simulink model "RCAM_OP_LONG_AP_SM_CL_FULL"  (R2022b)
settings: Solver=VariableStepAuto  StartTime=0.0  StopTime=100.0  RelTol=1e-3
undefined symbols (not defined in the file): H_nz, K_nzq
libraries: cstblocks x1
settings Model: Creator=bendr  LastModifiedBy=bendr

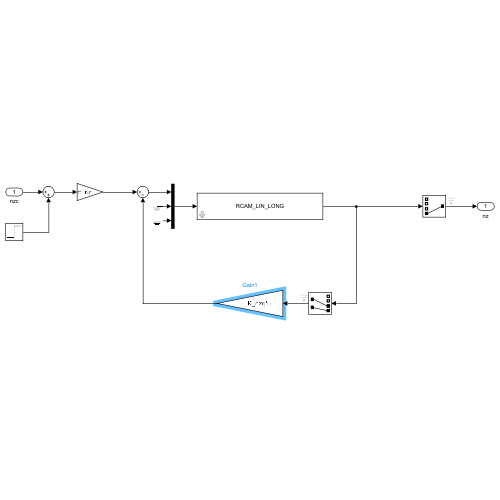
[thumbnail: Simulink's stored preview of the top-level diagram]
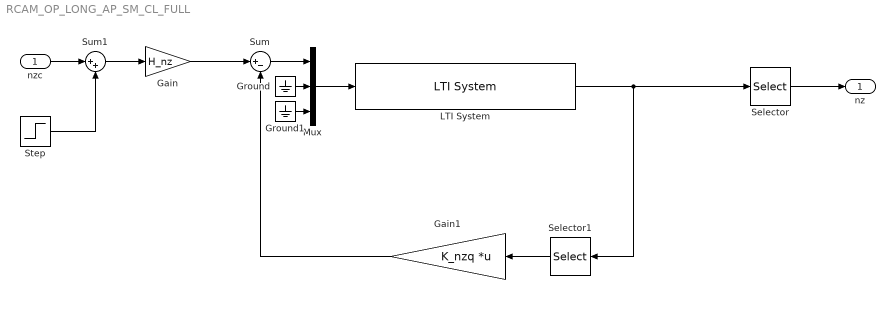
== system RCAM_OP_LONG_AP_SM_CL_FULL ==
  nzc : Inport
  Gain : Gain  Gain=H_nz
  Gain1 : Gain  Gain=K_nzq  Multiplication=Matrix(K*u)
  Ground : Ground
  Ground1 : Ground
  LTI System : cstblocks/LTI System  sys=RCAM_LIN_LONG  IC=[]
  Mux : Mux  Inputs=3
  Selector : Selector  InputPortWidth=4  IndexOptions=Index vector (dialog)  Indices=4  OutputSizes=1
  Selector1 : Selector  InputPortWidth=4  IndexOptions=Index vector (dialog)  Indices=[3 4]  OutputSizes=1
  Step : Step  SampleTime=0
  Sum : Sum  Inputs=|+-
  Sum1 : Sum  Inputs=|++
  nz : Outport
  wires:
  Gain/1 -> Sum/1
  Selector/1 -> nz/1
  LTI System/1 -> Selector1/1, Selector/1
  Gain1/1 -> Sum/2
  nzc/1 -> Sum1/1
  Sum1/1 -> Gain/1
  Step/1 -> Sum1/2
  Sum/1 -> Mux/1
  Mux/1 -> LTI System/1
  Ground/1 -> Mux/2
  Selector1/1 -> Gain1/1
  Ground1/1 -> Mux/3
